simulink model "mqtt_demo"  (R2025b)
settings: Solver=VariableStepAuto  StartTime=0.0  StopTime=inf  RelTol=1e-3
undefined symbols (not defined in the file or in its folder): reai, test
libraries: mqttlib x1
settings Model: Creator=SupachaiVorapojpisut  LastModifiedBy=IXVIA

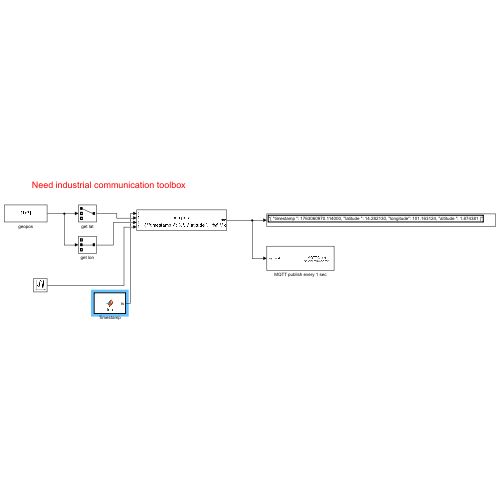
[thumbnail: Simulink's stored preview of the top-level diagram]
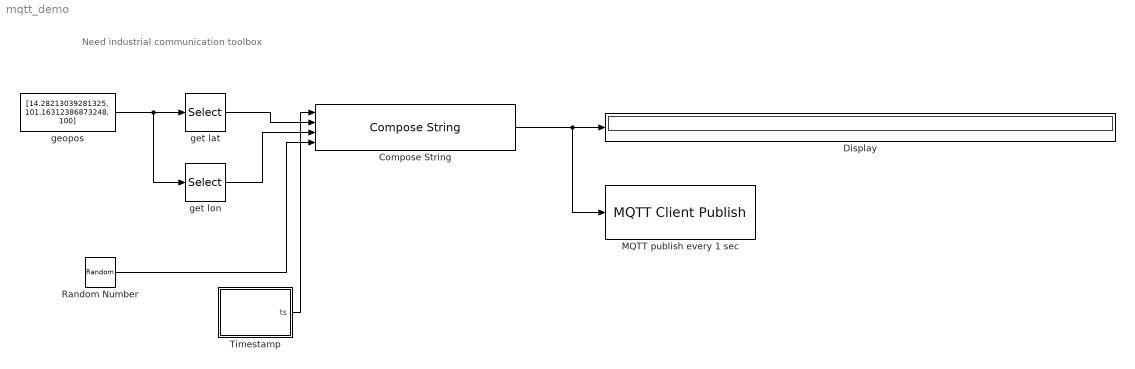
== system mqtt_demo ==
  note: Need industrial communication toolbox
  Compose String : ComposeString  Format="'{ \\\"timestamp \\\": %f, \\\"latitude \\\": %f, \\\"longitude\\\": %f, \\\"altitude \\\": %f }'"
  Display : Display
  MQTT publish every 1 sec : mqttlib/MQTT Client Publish  RetainClient=MQTTClient  ClientList=MQTTClient  TopicsTable={ '1', 'reai/test', '0', 'false' }  PublishOnDataChange=off  SampleTime=1  TopicNames=reai/test  NumTopics=1  IsLib=0  BlkName=MQTT Client Publish
  Random Number : RandomNumber  SampleTime=1
  Timestamp : MATLAB Function  TreatAsAtomicUnit=on
  geopos : Constant  Value=[14.28213039281325, 101.16312386873248, 100]
  get lat : Selector  InputPortWidth=3  IndexOptions=Index vector (dialog)  Indices=[1]  OutputSizes=1
  get lon : Selector  InputPortWidth=3  IndexOptions=Index vector (dialog)  Indices=[2]  OutputSizes=1
  wires:
  geopos/1 -> get lon/1, get lat/1
  get lat/1 -> Compose String/2
  get lon/1 -> Compose String/3
  Random Number/1 -> Compose String/4
  Compose String/1 -> MQTT publish every 1 sec/1, Display/1
  Timestamp/1(ts) -> Compose String/1

== matlab function mqtt_demo/Timestamp ==
  data: ts output
function ts = fcn()
    % Real-world UNIX timestamp
    ts = posixtime(datetime('now'));
end
